simulink model "vehicle_counting_serial"  (R2018b)
settings: Solver=VariableStepAuto  StartTime=0.0  StopTime=inf  RelTol=1e-3  EnableMultiTasking=on
undefined symbols (not defined in the file): gray, none, Rec, SDTV, serial, strel, videoinput
libraries: visiontextngfix x5, instrumentlib x2, visionstatistics x2, visionconversions x2, imaqlib x1, dspvision x1, visionmorphops x1, simulink x1
settings Model: Creator=Monty  LastModifiedBy=28122
settings DataIOCC: LimitDataPoints=on
settings OptimizationCC: LifeSpan=inf
settings DebuggingCC: AllowSymbolicDim=off  SFUnexpectedBacktrackingDiag=warning  SFNoUnconditionalDefaultTransitionDiag=warning  SFExecutionAtInitializationDiag=none
settings ModelReferenceCC: PropagateSignalLabelsOutOfModel=off
settings SFSimCC: SimUseLocalCustomCode=off
settings RTWCC: RTWUseLocalCustomCode=off
settings CodeAppCC: StateflowObjectComments=on
settings GRTTargetCC: TargetLangStandard=C89/C90 (ANSI)
settings ConfigComp: CovMetricSettings=dw  CovHtmlReporting=on  CovSaveCumulativeToWorkspaceVar=on  CovSaveSingleToWorkspaceVar=on  CovExternalEMLEnable=off

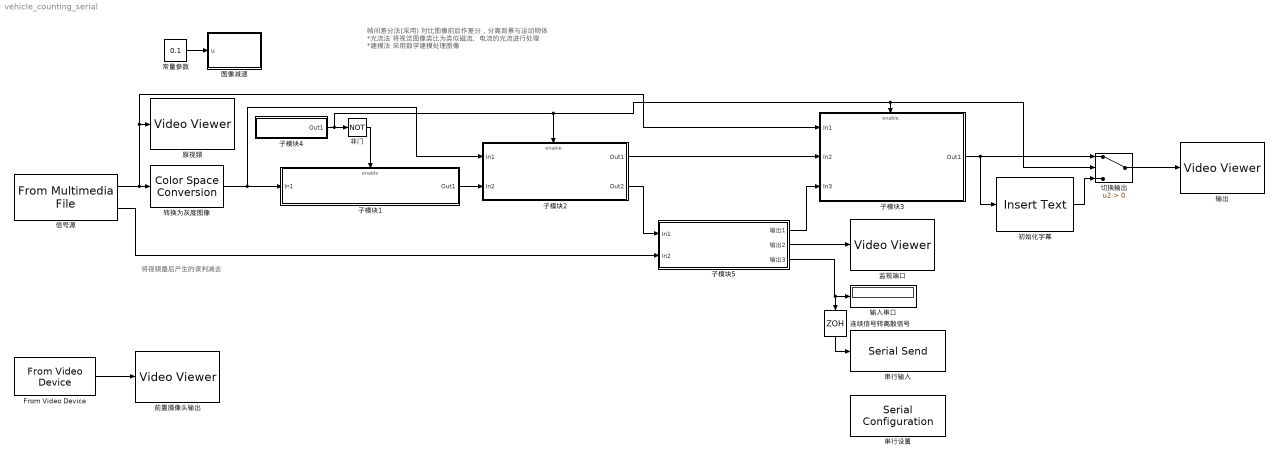
== system vehicle_counting_serial ==
  note: 将视频最后产生的误判减去
  note: 帧间差分法(采用)
      | 对比图像前后作差分，分离背景与运动物体
      | *光流法
      | 将视觉图像类比为类似磁流、电流的光流进行处理
      | *建模法
      | 采用数学建模处理图像
  From Video Device : imaqlib/From Video Device  DeviceMenu=winvideo 1 (Integrated Camera)  Device=winvideo 1 (Integrated Camera)  ObjConstructor=videoinput('winvideo', 1)  VideoFormatMenu=YUY2_320x240  VideoFormat=YUY2_320x240  VideoSource=input1  ROIPosition=[0 0 240 320]  EnableHWTrigger=off  TriggerConfiguration=none/none  SampleTime=1/15  OutputPortsMode=One multidimensional signal  DataType=single  CanDoHWTrigger=no  ReturnedColorSpace=rgb  BlockHandle=750.0004  ROIWidth=320  ROIHeight=240  ROIColumn=0  ROIRow=0  EngXMLPath=E:\Program Files (x86)\Matlab\toolbox\imaq\imaq\private  DevXMLPath=C:\ProgramData\MATLAB\SupportPackages\R2018b\toolbox\imaq\supportpackages\genericvideo\adaptor\win64  EngLibPath=E:\Program Files (x86)\Matlab\toolbox\imaq\imaqblks\imaqmex\win64  ColorSpace=rgb  BayerSensorAlignment=grbg
      settings: SourceProductName=Image Acquisition Toolbox
  串行设置 : instrumentlib/Serial Configuration  Priority=-200000  ComPortMenu=COM1  ComPort=COM1  ObjConstructor=serial('COM1');  BaudRate=9600  DataBits=8  Parity=none  StopBits=1  FlowControl=none  Timeout=10  ByteOrder=LittleEndian
  串行输入 : instrumentlib/Serial Send  ComPortMenu=COM1  ComPort=COM1  ObjConstructor=serial('COM1');  Terminator=<none>  EnableBlockingMode=on
  信号源 : dspvision/From Multimedia File  inputFilename=E:\Program Files (x86)\Matlab\toolbox\vision\visiondata\viptraffic.avi  loop=on  numPlays=inf  outputStreams=Video only  videoDataType=single  audioDataType=int16  inheritSampleTime=on  userDefinedSampleTime=1/30  noAudioOutput=off  isIntensityVideo=off  fourcc=RGB  colorVideoFormat=One multidimensional signal  outputEOF=on  dataOrg=Column-major  audioFrameSize=1024  computeAudioFrameSize=off  outSamplingMode=Sample based
      settings: SourceProductBaseCode=VP
  切换输出 : Switch  Criteria=u2 > Threshold
  初始化字幕 : visiontextngfix/Insert Text  inputType=Obsolete  theText='Initialing'  getTextLocFrom=Specify via dialog  textLoc=[50 50]  getTextColorFrom=Specify via dialog  textColor=[1 1 1]  getTextIntensityFrom=Specify via dialog  textIntensity=0  getTextOpacityFrom=Specify via dialog  textOpacity=1.0  dummyVar2=0  dummyVar3=0  dummyVar4=0  imagePorts=One multidimensional signal  isInputTransposed=off  fontFace=LucidaSansRegular  dummyVar1=0  blockFontSize=14  antiAliased=on
      settings: SourceProductName=Computer Vision System Toolbox  SourceProductBaseCode=VP
  前置摄像头输出 : VideoViewer  FigPos=[226.075630252101 499.781512605042 417.882352941176 304.134453781513]
  原视频 : VideoViewer  colormapValue=gray(256)  FigPos=[701 310 409.6 167.2]
  图像减速 : MATLAB Function  TreatAsAtomicUnit=on
  子模块1 : Subsystem
      mask Display:
      | disp('提取背景\n邱剑楠')
      | port_label('input',1,'原始视频输入口')
      | port_label('output',1,'背景图像')
  子模块2 : Subsystem
      mask Display:
      | disp('识别车辆\n邱剑楠')
      | port_label('input',1,'原始视频输入口')
      | port_label('input',2,'背景图像')
      | port_label('output',1,'位置')
      | port_label('output',2,'Blob图像')
  子模块3 : Subsystem
      mask Display:
      | disp('显示单元\n邱剑楠')
      | port_label('input',1,'原始视频输入口')
      | port_label('input',2,'位置信息')
      | port_label('input',3,'计数')
      | port_label('output',1,'结果输出')
  子模块4 : Subsystem
      mask Display:
      | disp('控制信号\n邱剑楠')
      | port_label('output',1,'')
  子模块5 : Subsystem
      mask Display:
      | disp('车辆计数\n信息1901_邱剑楠')
      | port_label('input',1,'Blob图像')
      | port_label('input',2,'EOF')
      | port_label('output',1,'车辆计数')
      | port_label('output',2,'监测端口')
      | port_label('output',3,'车流量')
  常量参数 : Constant  Value=0.1
  监视端口 : VideoViewer  colormapValue=gray(256)  FigPos=[277 304.4 409.6 167.2]
  转换为灰度图像 : visionconversions/Color Space  Conversion  conversion=Obsolete  conversionActive=R'G'B' to intensity  wp_str=D65  rec=Rec. 601 (SDTV)  sys=1125/60/2:1  imagePorts=One multidimensional signal
      settings: SourceProductName=Computer Vision System Toolbox
  输入串口 : Display
  输出 : VideoViewer  colormapValue=gray(256)  FigPos=[1132.02521008403 313.428571428571 409.81512605042 167.798319327731]
  连续信号转离散信号 : ZeroOrderHold  SampleTime=-1
  非门 : Logic  Operator=NOT  AllPortsSameDT=off  OutDataTypeStr=boolean
  wires:
  信号源/1 -> 子模块3/1(In1), 原视频/1, 转换为灰度图像/1
  子模块1/1(Out1) -> 子模块2/2(In2)
  子模块2/1(Out1) -> 子模块3/2(In2)
  子模块4/1(Out1) -> 子模块3/Enable, 切换输出/2, 子模块2/Enable, 非门/1
  非门/1 -> 子模块1/Enable
  转换为灰度图像/1 -> 子模块2/1(In1), 子模块1/1(In1)
  子模块3/1(Out1) -> 初始化字幕/1, 切换输出/1
  切换输出/1 -> 输出/1
  初始化字幕/1 -> 切换输出/3
  常量参数/1 -> 图像减速/1(u)
  子模块2/2(Out2) -> 子模块5/1(In1)
  信号源/2 -> 子模块5/2(In2)
  子模块5/2(输出2) -> 监视端口/1
  子模块5/3(输出3) -> 连续信号转离散信号/1, 输入串口/1
  子模块5/1(输出1) -> 子模块3/3(In3)
  From Video Device/1 -> 前置摄像头输出/1
  连续信号转离散信号/1 -> 串行输入/1

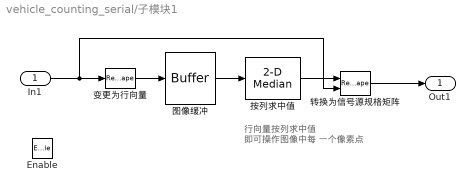
== system vehicle_counting_serial/子模块1 ==
  note: 行向量按列求中值
      | 即可操作图像中每
      | 一个像素点
  In1 : Inport
  Enable : EnablePort
  变更为行向量 : Reshape  OutputDimensionality=Row vector (2-D)
  图像缓冲 : Buffer  N=40  V=5  OutputFrames=off
  按列求中值 : visionstatistics/2-D Median  sortAlg=Quick sort  directionMode=Each column  dimension=1  treatSBRowAsCol=on  outputDataTypeStr=Inherit: Same as accumulator  outputLastDataTypeStr=Inherit: Same as accumulator  outputMin=[]  outputMax=[]  accumMode=Binary point scaling  accumWordLength=32  accumFracLength=0  accumDataTypeStr=fixdt([],32,0)  accumLastDataTypeStr=fixdt([],32,0)  roundingMode=Floor  overflowMode=off
      settings: SourceProductName=Computer Vision System Toolbox  SourceProductBaseCode=VP  allowOverrides=off
  转换为信号源规格矩阵 : Reshape  OutputDimensionality=Derive from reference input port
  Out1 : Outport
  wires:
  图像缓冲/1 -> 按列求中值/1
  按列求中值/1 -> 转换为信号源规格矩阵/1
  转换为信号源规格矩阵/1 -> Out1/1
  In1/1 -> 转换为信号源规格矩阵/2, 变更为行向量/1
  变更为行向量/1 -> 图像缓冲/1

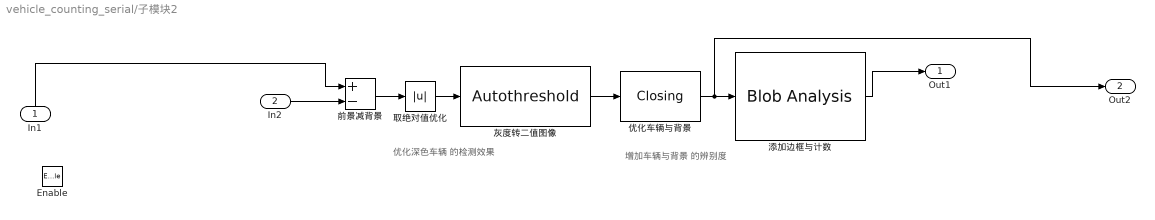
== system vehicle_counting_serial/子模块2 ==
  note: 增加车辆与背景
      | 的辨别度
  note: 优化深色车辆
      | 的检测效果
  In1 : Inport
  In2 : Inport  Port=2
  Enable : EnablePort
  优化车辆与背景 : visionmorphops/Closing  nhoodsrc=Specify via dialog  strel=strel('square',7)
      settings: SourceProductName=Computer Vision System Toolbox  SourceProductBaseCode=VP
  前景减背景 : Sum  Inputs=+-
  取绝对值优化 : Abs
  添加边框与计数 : visionstatistics/Blob Analysis  Tag=vipblks_row_conv  area=off  centroid=off  bBox=on  majorAxis=off  minorAxis=off  angle=off  eccentricity=off  equivDiameterSq=off  extent=off  perimeter=off  maxBlobs=10  warnIfNumBlobsExceeded=on  isCount=off  useMinArea=on  minArea=350  useMaxArea=on  maxArea=4000  excludeBorderBlob=off  outDT=double  isOutVarDim=off  isFill=on  fillValues=-1  conn=8  isLabel=off  outputMode=Binary point scaling  outputWordLength=32  outputFracLength=16  firstCoeffMode=Binary point scaling  firstCoeffWordLength=16  firstCoeffFracLength=14  secondCoeffMode=Binary point scaling  secondCoeffWordLength=32  secondCoeffFracLength=16  accumMode=Binary point scaling  accumWordLength=32  accumFracLength=0  prodOutputMode=Binary point scaling  prodOutputWordLength=32  prodOutputFracLength=16  roundingMode=Floor  overflowMode=off
      settings: SourceProductName=Computer Vision System Toolbox
  灰度转二值图像 : visionconversions/Autothreshold  operator=>  threshOut=off  effMetricOut=off  userDefinedRange=off  umin=0  umax=255  outOfRngOpt=Warn and saturate  scaleThreshold=off  scaleFactor=1  P1Mode=Specify word length  P1WordLength=32  P1FracLength=30  P2Mode=Specify word length  P2WordLength=32  P2FracLength=22  P3Mode=Specify word length  P3WordLength=32  P3FracLength=14  P4Mode=Binary point scaling  P4WordLength=32  P4FracLength=15  Q1Mode=Specify word length  Q1WordLength=32  Q1FracLength=16  EMMode=Specify word length  EMWordLength=16  EMFracLength=14  roundingMode=Floor  overflowMode=off
      settings: SourceProductName=Computer Vision System Toolbox  SourceProductBaseCode=VP
  Out1 : Outport
  Out2 : Outport  Port=2
  wires:
  添加边框与计数/1 -> Out1/1
  取绝对值优化/1 -> 灰度转二值图像/1
  In1/1 -> 前景减背景/1
  灰度转二值图像/1 -> 优化车辆与背景/1
  优化车辆与背景/1 -> Out2/1, 添加边框与计数/1
  In2/1 -> 前景减背景/2
  前景减背景/1 -> 取绝对值优化/1

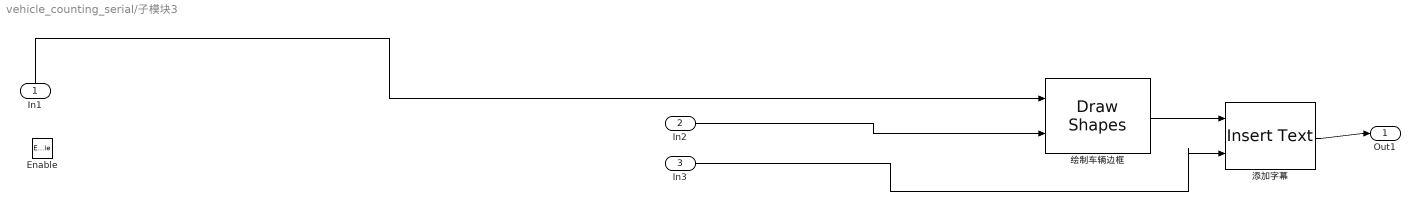
== system vehicle_counting_serial/子模块3 ==
  In1 : Inport
  In2 : Inport  Port=2
  In3 : Inport  Port=3
  Enable : EnablePort
  添加字幕 : visiontextngfix/Insert Text  inputType=Obsolete  theText='%3d car are found'  getTextLocFrom=Specify via dialog  textLoc=[10 6]  getTextColorFrom=Specify via dialog  textColor=[1 1 1]  getTextIntensityFrom=Specify via dialog  textIntensity=0  getTextOpacityFrom=Specify via dialog  textOpacity=1.0  dummyVar2=0  dummyVar3=0  dummyVar4=0  imagePorts=One multidimensional signal  isInputTransposed=off  fontFace=LucidaSansRegular  dummyVar1=0  blockFontSize=14  antiAliased=on
      settings: SourceProductName=Computer Vision System Toolbox  SourceProductBaseCode=VP
  绘制车辆边框 : visiontextngfix/Draw Shapes  shape=Rectangles  fill=off  lineWidth=2  fillClrSource=Specify via dialog  display=User-specified value  intensity=200  color=[0 0 1]  opacity=0.6  viewport=Entire image  antialiasing=off  inType=Obsolete  imagePorts=One multidimensional signal  prodOutputMode=Binary point scaling  prodOutputWordLength=32  prodOutputFracLength=14  memoryMode=Specify word length  memoryWordLength=16  memoryFracLength=15  roundingMode=Floor  overflowMode=off
      settings: SourceProductName=Computer Vision System Toolbox
  Out1 : Outport
  wires:
  添加字幕/1 -> Out1/1
  In2/1 -> 绘制车辆边框/2
  In3/1 -> 添加字幕/2
  绘制车辆边框/1 -> 添加字幕/1
  In1/1 -> 绘制车辆边框/1

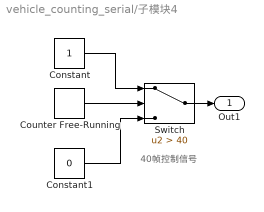
== system vehicle_counting_serial/子模块4 ==
  note: 40帧控制信号
  Constant : Constant
  Constant1 : Constant  Value=0
  Counter Free-Running : simulink/Sources/Counter Free-Running  NumBits=16  tsamp=1/15
  Switch : Switch  Criteria=u2 > Threshold  Threshold=40
  Out1 : Outport
  wires:
  Constant/1 -> Switch/1
  Counter Free-Running/1 -> Switch/2
  Constant1/1 -> Switch/3
  Switch/1 -> Out1/1

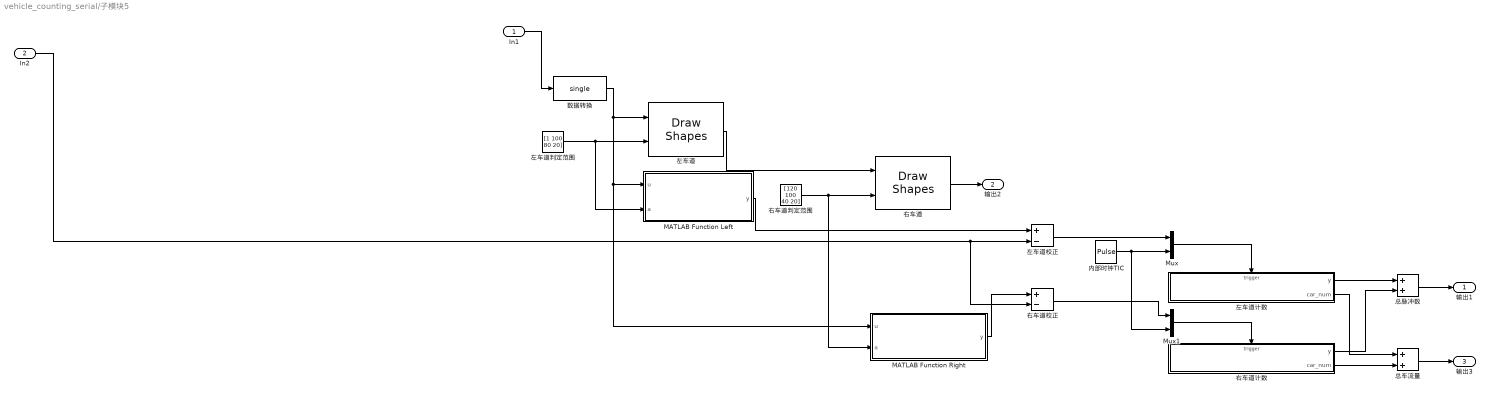
== system vehicle_counting_serial/子模块5 ==
  In1 : Inport
  In2 : Inport  Port=2
  MATLAB Function Left : MATLAB Function  TreatAsAtomicUnit=on
  MATLAB Function Right : MATLAB Function  TreatAsAtomicUnit=on
  Mux : Mux  Inputs=2
  Mux1 : Mux  Inputs=2
  内部时钟TIC : DiscretePulseGenerator  PulseType=Time based  Period=1  PulseWidth=50
  右车道 : visiontextngfix/Draw Shapes  shape=Rectangles  fill=on  lineWidth=2  fillClrSource=Specify via dialog  display=White  intensity=200  color=[200 255 100]  opacity=0.6  viewport=Entire image  antialiasing=off  inType=Obsolete  imagePorts=One multidimensional signal  prodOutputMode=Binary point scaling  prodOutputWordLength=32  prodOutputFracLength=14  memoryMode=Specify word length  memoryWordLength=16  memoryFracLength=14  roundingMode=Floor  overflowMode=off
      settings: SourceProductName=Computer Vision System Toolbox
  右车道判定范围 : Constant  Value=[120 100 40 20]
  右车道校正 : Sum  Inputs=+-
  右车道计数 : Stateflow chart  TreatAsAtomicUnit=on
  左车道 : visiontextngfix/Draw Shapes  shape=Rectangles  fill=on  lineWidth=2  fillClrSource=Specify via dialog  display=White  intensity=200  color=[200 255 100]  opacity=0.6  viewport=Entire image  antialiasing=off  inType=Obsolete  imagePorts=One multidimensional signal  prodOutputMode=Binary point scaling  prodOutputWordLength=32  prodOutputFracLength=14  memoryMode=Specify word length  memoryWordLength=16  memoryFracLength=14  roundingMode=Floor  overflowMode=off
      settings: SourceProductName=Computer Vision System Toolbox
  左车道判定范围 : Constant  Value=[1 100 80 20]
  左车道校正 : Sum  Inputs=+-
  左车道计数 : Stateflow chart  TreatAsAtomicUnit=on
  总脉冲数 : Sum  OutDataTypeStr=int16
  总车流量 : Sum  OutDataTypeStr=int16
  数据转换 : DataTypeConversion  OutDataTypeStr=single
  输出1 : Outport
  输出2 : Outport  Port=2
  输出3 : Outport  Port=3
  wires:
  内部时钟TIC/1 -> Mux1/2, Mux/2
  Mux/1 -> 左车道计数/Trigger
  右车道计数/1(y) -> 总脉冲数/2
  左车道计数/1(y) -> 总脉冲数/1
  In1/1 -> 数据转换/1
  数据转换/1 -> MATLAB Function Right/1(u), MATLAB Function Left/1(u), 左车道/1
  左车道/1 -> 右车道/1
  左车道判定范围/1 -> MATLAB Function Left/2(a), 左车道/2
  右车道/1 -> 输出2/1
  In2/1 -> 右车道校正/2, 左车道校正/2
  MATLAB Function Right/1(y) -> 右车道校正/1
  右车道判定范围/1 -> MATLAB Function Right/2(a), 右车道/2
  MATLAB Function Left/1(y) -> 左车道校正/1
  左车道校正/1 -> Mux/1
  Mux1/1 -> 右车道计数/Trigger
  右车道校正/1 -> Mux1/1
  左车道计数/2(car_num) -> 总车流量/1
  右车道计数/2(car_num) -> 总车流量/2
  总脉冲数/1 -> 输出1/1
  总车流量/1 -> 输出3/1

== matlab function vehicle_counting_serial/子模块5/MATLAB Function Left ==
  data: u input; y output; a input
function y = fcn(u,a)
%#codegen
  
auto1=0;	%初始化变量

ind_ant1=0;	%初始化变量

diferencia=zeros(size(u,1),size(u,2));%定义与图像u大小相同的空白图像                       
                                       %diferencia
for f=a(2):(a(2)+a(4))	%将输入图像u对应区域a中的内容复制到diferencia中
    for c=a(1):a(1)+a(3)
       diferencia(f,c)=u(f,c) ;
    end
end


[i j]=find(diferencia==1);%将diferencia中值为1的像素点找出来
fc=[i j];	%放入fc中
if  isempty(fc)	%若fc为空，将ind1设置为0
    ind1=0;
else			%若fc不为空，将ind1设置为1
    ind1=1;
end
 if ind_ant1==0 && ind1==1		%设置输出变量auto1
        auto1=auto1+1;           
    end
    ind_ant1=ind1;
y = auto1;

== matlab function vehicle_counting_serial/图像减速 ==
  data: u input
function fcn(u)
%#codegen

pause(u);

== matlab function vehicle_counting_serial/子模块5/MATLAB Function Right ==
  data: u input; y output; a input
function y = fcn(u,a)
%#codegen
  
auto1=0;	%初始化变量

ind_ant1=0;	%初始化变量

diferencia=zeros(size(u,1),size(u,2));%定义与图像u大小相同的空白图像                       
                                       %diferencia
for f=a(2):(a(2)+a(4))	%将输入图像u对应区域a中的内容复制到diferencia中
    for c=a(1):a(1)+a(3)
       diferencia(f,c)=u(f,c) ;
    end
end


[i j]=find(diferencia==1);%将diferencia中值为1的像素点找出来
fc=[i j];	%放入fc中
if  isempty(fc)	%若fc为空，将ind1设置为0
    ind1=0;
else			%若fc不为空，将ind1设置为1
    ind1=1;
end
 if ind_ant1==0 && ind1==1		%设置输出变量auto1
        auto1=auto1+1;           
    end
    ind_ant1=ind1;
y = auto1;

== stateflow chart vehicle_counting_serial/子模块5/左车道计数 ==
  state Main [parallel]
    settings: executionOrder=1
    state Reset
      entry:y=0;
      Timeout=0;
      Count=0;
    state Running
      entry:y=y+1;
    (default) -> Reset
    (junction 5) -> Running [order 2] : [Timeout==0]
    Reset -> Running : Pulse
    (junction 5) -> Reset [order 1] : [Timeout==1]/{car_num=y;}
    Running -> (junction 5) : Pulse
  state Timing [parallel]
    settings: executionOrder=2
    Timing -> (junction 15) : TIC
    (junction 15) -> (junction 17) [order 1] : [Count>99]
    (junction 15) -> (junction 21) [order 2] : {Count=Count+1;}
    (junction 17) -> (junction 19) : {Timeout=1;}
    (junction 19) -> (junction 21)
    (junction 21) -> (junction 24)
  data: y output; Count local; Timeout local; car_num output
  events: Pulse input RISING_EDGE_EVENT; TIC input RISING_EDGE_EVENT

== stateflow chart vehicle_counting_serial/子模块5/右车道计数 ==
  state Main [parallel]
    settings: executionOrder=1
    state Reset
      entry:y=0;
      Timeout=0;
      Count=0;
    state Running
      entry:y=y+1;
    (default) -> Reset
    (junction 5) -> Running [order 2] : [Timeout==0]
    Reset -> Running : Pulse
    (junction 5) -> Reset [order 1] : [Timeout==1]/{car_num=y;}
    Running -> (junction 5) : Pulse
  state Timing [parallel]
    settings: executionOrder=2
    Timing -> (junction 15) : TIC
    (junction 15) -> (junction 17) [order 1] : [Count>99]
    (junction 15) -> (junction 21) [order 2] : {Count=Count+1;}
    (junction 17) -> (junction 19) : {Timeout=1;}
    (junction 19) -> (junction 21)
    (junction 21) -> (junction 24)
  data: y output; Count local; Timeout local; car_num output
  events: Pulse input RISING_EDGE_EVENT; TIC input RISING_EDGE_EVENT
